simulink model "Proyecto_Final"  (R2017a)
settings: Solver=ode45  StartTime=0.0  StopTime=inf  FixedStep=0.002  RelTol=1e-4
values from neighbouring files (symbols this model uses):
  b_h = b_eq_h * r_h ^ 2 / R_d ^ 2    (= 28800)    [automatas_matlab.m]
  b_t = b_eq_t * r_t ^ 2 / R_w_t ^ 2    (= 27000)    [automatas_matlab.m]
  b_w_h = 30000    [automatas_matlab.m]
  ba_h = M_h * n_h * w_pos_h    (= 172800)    [automatas_matlab.m]
  ba_t = M_t * n_t * w_pos_t    (= 135000)    [automatas_matlab.m]
  bottom_limit_0 = -22    [automatas_matlab.m]
  bottom_limit_1 = -20    [automatas_matlab.m]
  container_vector = [2, 6, 4, 1, 5, 8, 1, 3, 7, 1, 5, 6]    [automatas_matlab.m]    (also in plot_crane.m = [8, 12, 12, 4, 5, 8, 1, 3]; test_traj.m = [8, 5, 9, 4, 5, 8, 4, 6]; test_trajectories.m = [8, 12, 12, 4, 5, 8, 1, 3, 7, 1, 5, 6])
  g = 9.80665    [automatas_matlab.m]
  h_contenedor = 2.79    [automatas_matlab.m]
  K_w_h = 1800000    [automatas_matlab.m]
  Ksa_h = M_h * n_h * w_pos_h^2    (= 207298.578199)    [automatas_matlab.m]
  Ksa_t = M_t * n_t * w_pos_t^2    (= 123542.570499)    [automatas_matlab.m]
  Ksia_h = M_h * w_pos_h ^ 3    (= 82894.8698367)    [automatas_matlab.m]
  Ksia_t = M_t * w_pos_t ^ 3    (= 45223.0125199)    [automatas_matlab.m]
  lambda = 0.91    [automatas_matlab.m]
  left_limit_0 = -32    [automatas_matlab.m]
  left_limit_1 = -30    [automatas_matlab.m]
  M_h = (J_d + J_m_h * r_h ^ 2)/ R_d ^ 2    (= 48014.2222222)    [automatas_matlab.m]
  m_l = 65000    [automatas_matlab.m]
  m_l_min = 15000    [automatas_matlab.m]
  M_t = m_c + (J_w_t + J_m_t * r_t ^ 2)/ R_w_t ^ 2    (= 59008)    [automatas_matlab.m]
  R_d = 0.75    [automatas_matlab.m]
  r_h = 30    [automatas_matlab.m]
  r_t = 15    [automatas_matlab.m]
  R_w_t = 0.5    [automatas_matlab.m]
  right_limit_0 = 52    [automatas_matlab.m]
  right_limit_1 = 50    [automatas_matlab.m]
  top_limit_0 = 42    [automatas_matlab.m]
  top_limit_1 = 40    [automatas_matlab.m]
  v_max_h_load = 1.5    [automatas_matlab.m]
  v_max_h_unload = 3    [automatas_matlab.m]
  v_max_t = 4    [automatas_matlab.m]
  x_t0 = 0    [automatas_matlab.m]
  y_t0 = 45    [automatas_matlab.m]    (also in crane.m; plot_crane.m; plot_crane_test.m)
  yl0 = h_contenedor + 5    (= 7.79)    [automatas_matlab.m]
undefined symbols (not defined in the file or in its folder): DiscIntNeverNeededParam
libraries: simulink x8, vrlib x1, sldrtlib x1
(part 1 of 2)
settings Model: SimulationMode=accelerator  Creator=elust  LastModifiedBy=laure
settings OptimizationCC: UseDivisionForNetSlopeComputation=on  UseFloatMulNetSlope=on  DefaultUnderspecifiedDataType=single  StateBitsets=on  DataBitsets=on  EfficientMapNaN2IntZero=off
settings HardwareCC: TargetBitPerPointer=64  TargetBitPerSizeT=64  TargetBitPerPtrDiffT=64  TargetLongLongMode=on  TargetIntDivRoundTo=Zero  TargetEndianess=LittleEndian  TargetWordSize=64  TargetHWDeviceType=MATLAB Host  ProdEqTarget=off
settings CodeAppCC: MaxIdLength=128
settings GRTTargetCC: TargetLangStandard=C89/C90 (ANSI)  CombineOutputUpdateFcns=off  GRTInterface=on

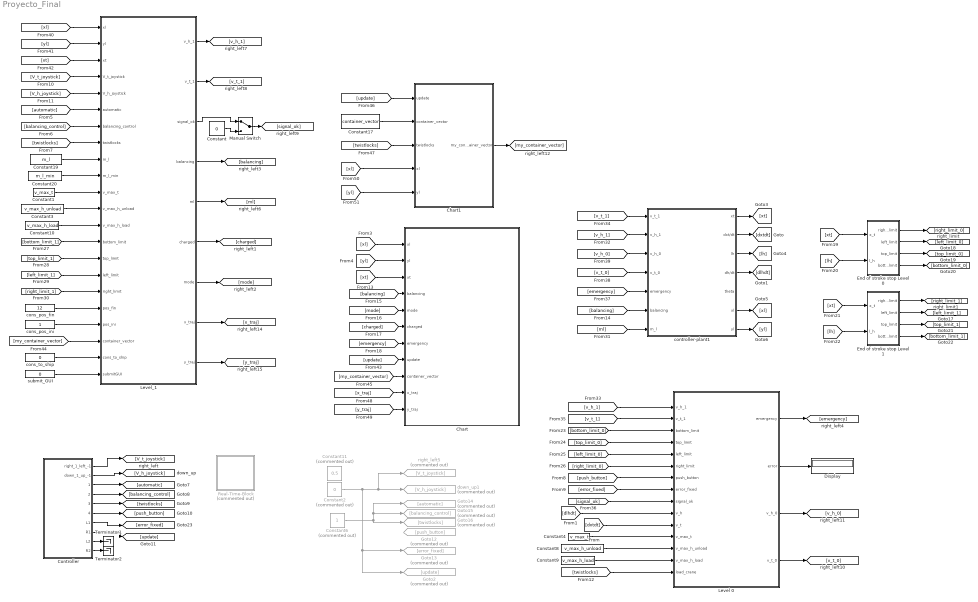
== system Proyecto_Final ==
  Chart : Stateflow chart  TreatAsAtomicUnit=on
  Chart1 : Stateflow chart  TreatAsAtomicUnit=on
  Constant : Constant  Value=0
  Constant1 : Constant  Value=v_max_t
  Constant10 : Constant  Value=v_max_h_load
  Constant11 : Constant  Commented=on  Value=0.5
  Constant17 : Constant  Value=container_vector
  Constant19 : Constant  Value=m_l
  Constant2 : Constant  Commented=on  Value=0
  Constant20 : Constant  Value=m_l_min
  Constant3 : Constant  Value=v_max_h_unload
  Constant4 : Constant  Value=v_max_t
  Constant6 : Constant  Commented=on
  Constant8 : Constant  Value=v_max_h_unload
  Constant9 : Constant  Value=v_max_h_load
  Controller : Subsystem
  Display : Display
  End of stroke stop Level 0 : Subsystem
  End of stroke stop Level 1 : Subsystem
  Goto12 : Goto  Commented=on  GotoTag=push_button
  Goto13 : Goto  Commented=on  GotoTag=error_fixed
  Goto14 : Goto  Commented=on  GotoTag=automatic
  Goto15 : Goto  Commented=on  GotoTag=balancing_control
  Goto16 : Goto  Commented=on  GotoTag=twistlocks
  Goto2 : Goto  Commented=on  GotoTag=update
  Level 0 : Stateflow chart  TreatAsAtomicUnit=on
  "Level_1 " : Stateflow chart  TreatAsAtomicUnit=on
  Manual Switch : ManualSwitch
  Real-Time-Block : Subsystem  Commented=on
  Terminator1 : Terminator
  Terminator2 : Terminator
  cons_pos_fin : Constant  Value=12
  cons_pos_ini : Constant
  cons_to_ship : Constant  Value=0
  controller-plant1 : Subsystem
  down_up1 : Goto  Commented=on  GotoTag=V_h_joystick
  right_left5 : Goto  Commented=on  GotoTag=V_t_joystick
  submit_GUI : Constant  Value=0
  wires:
  Level 0/2(error) -> Display/1
  [push_button] -> Level 0/7(push_button)
  [error_fixed] -> Level 0/8(error_fixed)
  Constant4/1 -> Level 0/12(v_max_t)
  Constant8/1 -> Level 0/13(v_max_h_unload)
  Constant9/1 -> Level 0/14(v_max_h_load)
  [twistlocks] -> Level 0/15(load_crane)
  controller-plant1/2(dxt/dt) -> [dxtdt]
  [dxtdt] -> Level 0/11(v_t)
  [dlhdt] -> Level 0/10(v_h)
  controller-plant1/4(dh/dt) -> [dlhdt]
  controller-plant1/1("xt ") -> [xt]
  controller-plant1/3(lh) -> [lh]
  controller-plant1/6(xl) -> [xl]
  controller-plant1/7(yl) -> [yl]
  Level 0/4(v_t_0) -> [v_t_0]
  Constant/1 -> Manual Switch/2
  "Level_1 "/3(signal_ok) -> Manual Switch/1
  Level 0/1(emergency) -> [emergency]
  Level 0/3(v_h_0) -> [v_h_0]
  Constant19/1 -> "Level_1 "/9(m_l)
  Constant20/1 -> "Level_1 "/10(m_l_min)
  Controller/3(1) -> [automatic]
  Controller/4(2) -> [balancing_control]
  Controller/5(3) -> [twistlocks]
  Controller/6(4) -> [push_button]
  [automatic] -> "Level_1 "/6(automatic)
  [balancing_control] -> "Level_1 "/7(balancing_control)
  [twistlocks] -> "Level_1 "/8(twistlocks)
  Controller/8(R1) -> [update]
  Controller/1(right_1_left_-1) -> [V_t_joystick]
  Controller/2(down_1_up_-1) -> [V_h_joystick]
  Controller/7(L1) -> [error_fixed]
  Controller/9(L2) -> Terminator1/1
  Controller/10(R2) -> Terminator2/1
  [V_t_joystick] -> "Level_1 "/4(V_t_joystick)
  [V_h_joystick] -> "Level_1 "/5(V_h_joystick)
  [yl] -> Chart/2(yl)
  [xl] -> Chart/1(xl)
  Constant1/1 -> "Level_1 "/11(v_max_t)
  Constant3/1 -> "Level_1 "/12(v_max_h_unload)
  Constant10/1 -> "Level_1 "/13(v_max_h_load)
  [xt] -> Chart/3(xt)
  "Level_1 "/7(mode) -> [mode]
  "Level_1 "/6(charged) -> [charged]
  "Level_1 "/4(balancing) -> [balancing]
  [balancing] -> controller-plant1/6(balancing)
  [charged] -> Chart/6(charged)
  [mode] -> Chart/5(mode)
  [balancing] -> Chart/4(balancing)
  [emergency] -> Chart/7(emergency)
  [xt] -> End of stroke stop Level 0/1(x_t)
  [lh] -> End of stroke stop Level 0/2(l_h)
  End of stroke stop Level 0/1(right_limit) -> [right_limit_0]
  End of stroke stop Level 0/2(left_limit) -> [left_limit_0]
  End of stroke stop Level 0/3(top_limit) -> [top_limit_0]
  End of stroke stop Level 0/4(bottom_limit) -> [bottom_limit_0]
  [lh] -> End of stroke stop Level 1/2(l_h)
  [xt] -> End of stroke stop Level 1/1(x_t)
  [right_limit_0] -> Level 0/6(right_limit)
  [left_limit_0] -> Level 0/5(left_limit)
  [top_limit_0] -> Level 0/4(top_limit)
  [bottom_limit_0] -> Level 0/3(bottom_limit)
  End of stroke stop Level 1/4(bottom_limit) -> [bottom_limit_1]
  End of stroke stop Level 1/3(top_limit) -> [top_limit_1]
  End of stroke stop Level 1/2(left_limit) -> [left_limit_1]
  End of stroke stop Level 1/1(right_limit) -> [right_limit_1]
  [bottom_limit_1] -> "Level_1 "/14(bottom_limit)
  [top_limit_1] -> "Level_1 "/15(top_limit)
  [left_limit_1] -> "Level_1 "/16(left_limit)
  [right_limit_1] -> "Level_1 "/17(right_limit)
  "Level_1 "/5(ml) -> [ml]
  [ml] -> controller-plant1/7(m_l)
  [v_h_1] -> controller-plant1/2(v_h_1)
  [v_h_1] -> Level 0/1(v_h_1)
  "Level_1 "/1(v_h_1) -> [v_h_1]
  "Level_1 "/2(v_t_1) -> [v_t_1]
  [v_t_1] -> controller-plant1/1(v_t_1)
  [v_t_1] -> Level 0/2(v_t_1)
  Manual Switch/1 -> [signal_ok]
  [signal_ok] -> Level 0/9(signal_ok)
  [emergency] -> controller-plant1/5(emergency)
  [v_t_0] -> controller-plant1/4(v_t_0)
  [v_h_0] -> controller-plant1/3(v_h_0)
  cons_pos_fin/1 -> "Level_1 "/18(pos_fin)
  cons_pos_ini/1 -> "Level_1 "/19(pos_ini)
  [xt] -> "Level_1 "/3(xt)
  [yl] -> "Level_1 "/2(yl)
  [xl] -> "Level_1 "/1(xl)
  [update] -> Chart/8(update)
  Chart1/1(my_container_vector) -> [my_container_vector]
  Constant17/1 -> Chart1/2(container_vector)
  [my_container_vector] -> "Level_1 "/20(container_vector)
  [my_container_vector] -> Chart/9(container_vector)
  [update] -> Chart1/1(update)
  [twistlocks] -> Chart1/3(twistlocks)
  "Level_1 "/9(y_traj) -> [y_traj]
  "Level_1 "/8(x_traj) -> [x_traj]
  [x_traj] -> Chart/10(x_traj)
  [y_traj] -> Chart/11(y_traj)
  [xl] -> Chart1/4(xl)
  cons_to_ship/1 -> "Level_1 "/21(cons_to_ship)
  submit_GUI/1 -> "Level_1 "/22(submitGUI)
  [yl] -> Chart1/5(yl)
  Constant2/1 -> Goto13/1, Goto2/1, right_left5/1, down_up1/1
  Constant6/1 -> Goto15/1, Goto14/1, Goto16/1

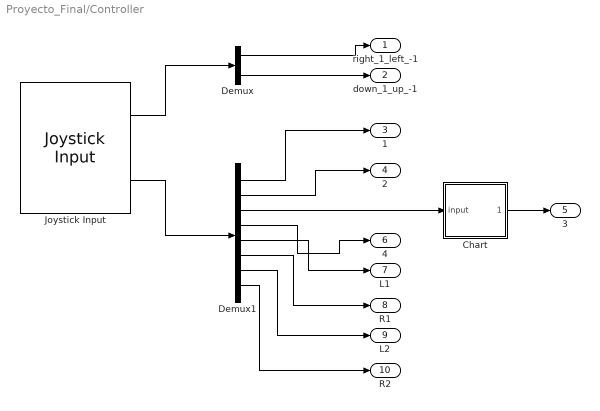
== system Proyecto_Final/Controller ==
  Chart : Stateflow chart  TreatAsAtomicUnit=on
  Demux : Demux  Outputs=2
  Demux1 : Demux  Outputs=8
  Joystick Input : vrlib/Joystick Input  joyid=1  adjustports=on  forcefeed=off
      settings: SourceProductBaseCode=VR
  right_1_left_-1 : Outport
  down_1_up_-1 : Outport  Port=2
  1 : Outport  Port=3
  2 : Outport  Port=4
  3 : Outport  Port=5
  4 : Outport  Port=6
  L1 : Outport  Port=7
  R1 : Outport  Port=8
  L2 : Outport  Port=9
  R2 : Outport  Port=10
  wires:
  Joystick Input/1 -> Demux/1
  Joystick Input/2 -> Demux1/1
  Demux1/1 -> 1/1
  Demux1/2 -> 2/1
  Demux1/8 -> R2/1
  Demux1/5 -> L1/1
  Demux1/4 -> 4/1
  Demux/1 -> right_1_left_-1/1
  Demux1/6 -> R1/1
  Demux1/7 -> L2/1
  Demux/2 -> down_1_up_-1/1
  Demux1/3 -> Chart/1(input)
  Chart/1(output) -> 3/1

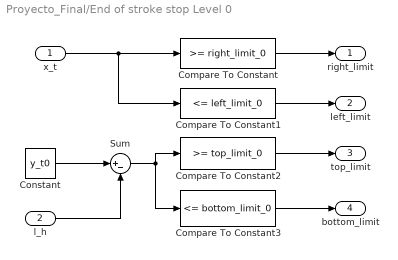
== system Proyecto_Final/End of stroke stop Level 0 ==
  x_t : Inport
  l_h : Inport  Port=2
  Compare To Constant : simulink/Logic and Bit Operations/Compare To Constant  relop=>=  const=right_limit_0  OutDataTypeStr=boolean
  Compare To Constant1 : simulink/Logic and Bit Operations/Compare To Constant  relop=<=  const=left_limit_0  OutDataTypeStr=boolean
  Compare To Constant2 : simulink/Logic and Bit Operations/Compare To Constant  relop=>=  const=top_limit_0  OutDataTypeStr=boolean
  Compare To Constant3 : simulink/Logic and Bit Operations/Compare To Constant  relop=<=  const=bottom_limit_0  OutDataTypeStr=boolean
  Constant : Constant  Value=y_t0
  Sum : Sum  Inputs=|+-
  right_limit : Outport
  left_limit : Outport  Port=2
  top_limit : Outport  Port=3
  bottom_limit : Outport  Port=4
  wires:
  Compare To Constant3/1 -> bottom_limit/1
  Compare To Constant1/1 -> left_limit/1
  Compare To Constant/1 -> right_limit/1
  Compare To Constant2/1 -> top_limit/1
  x_t/1 -> Compare To Constant1/1, Compare To Constant/1
  Constant/1 -> Sum/1
  l_h/1 -> Sum/2
  Sum/1 -> Compare To Constant2/1, Compare To Constant3/1

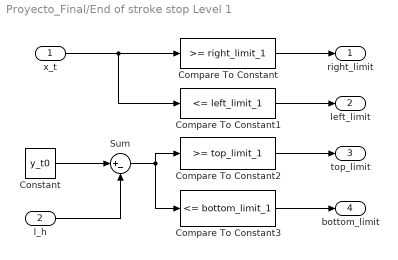
== system Proyecto_Final/End of stroke stop Level 1 ==
  x_t : Inport
  l_h : Inport  Port=2
  Compare To Constant : simulink/Logic and Bit Operations/Compare To Constant  relop=>=  const=right_limit_1  OutDataTypeStr=boolean
  Compare To Constant1 : simulink/Logic and Bit Operations/Compare To Constant  relop=<=  const=left_limit_1  OutDataTypeStr=boolean
  Compare To Constant2 : simulink/Logic and Bit Operations/Compare To Constant  relop=>=  const=top_limit_1  OutDataTypeStr=boolean
  Compare To Constant3 : simulink/Logic and Bit Operations/Compare To Constant  relop=<=  const=bottom_limit_1  OutDataTypeStr=boolean
  Constant : Constant  Value=y_t0
  Sum : Sum  Inputs=|+-
  right_limit : Outport
  left_limit : Outport  Port=2
  top_limit : Outport  Port=3
  bottom_limit : Outport  Port=4
  wires:
  Compare To Constant3/1 -> bottom_limit/1
  Compare To Constant1/1 -> left_limit/1
  Compare To Constant/1 -> right_limit/1
  Compare To Constant2/1 -> top_limit/1
  x_t/1 -> Compare To Constant1/1, Compare To Constant/1
  Constant/1 -> Sum/1
  l_h/1 -> Sum/2
  Sum/1 -> Compare To Constant2/1, Compare To Constant3/1

== system Proyecto_Final/Real-Time-Block ==
  Missed Ticks : Scope
  Real-Time Synchronization : sldrtlib/Real-Time Synchronization  SampleTime=0.1  MaxMissedTicks=10000  ShowMissedTicks=on  YieldWhenWaiting=off
  wires:
  Real-Time Synchronization/1 -> Missed Ticks/1

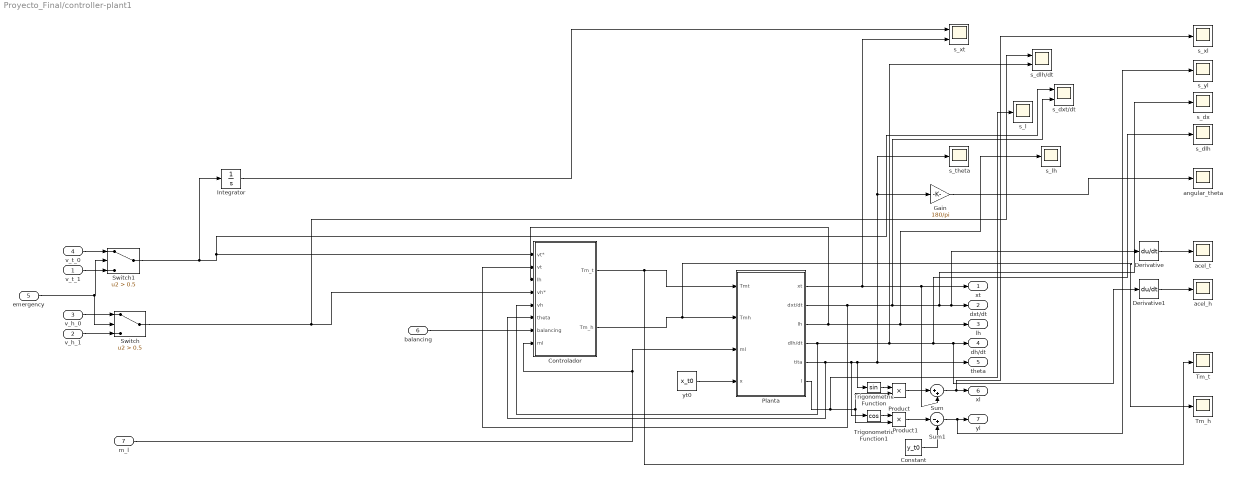
== system Proyecto_Final/controller-plant1 ==
  v_t_1 : Inport
  v_h_1 : Inport  Port=2
  v_h_0 : Inport  Port=3
  v_t_0 : Inport  Port=4
  emergency : Inport  Port=5
  balancing : Inport  Port=6
  m_l : Inport  Port=7
  Constant : Constant  Value=y_t0
  Controlador : Subsystem
  Derivative : Derivative
  Derivative1 : Derivative
  Gain : Gain  Gain=180/pi
  Integrator : Integrator
  Planta : Subsystem
  Product : Product
  Product1 : Product
  Sum : Sum  Inputs=|++
  Sum1 : Sum  Inputs=|-+
  Switch : Switch  Criteria=u2 > Threshold  Threshold=0.5
  Switch1 : Switch  Criteria=u2 > Threshold  Threshold=0.5
  Tm_h : Scope
  "Tm_t " : Scope
  Trigonometric Function : Trigonometry
  Trigonometric Function1 : Trigonometry  Operator=cos
  acel_h : Scope
  acel_t : Scope
  angular_theta : Scope
  s_dlh : Scope
  s_dlh/dt : Scope  NumInputPorts=2
  s_dx : Scope
  s_dxt/dt : Scope  NumInputPorts=2
  s_l : Scope
  s_lh : Scope
  "s_theta " : Scope
  "s_xl " : Scope
  s_xt : Scope  NumInputPorts=2
  "s_yl " : Scope
  yt0 : Constant  Value=x_t0
  "xt " : Outport
  dxt/dt : Outport  Port=2
  lh : Outport  Port=3
  dh/dt : Outport  Port=4
  theta : Outport  Port=5
  xl : Outport  Port=6
  yl : Outport  Port=7
  wires:
  Switch1/1 -> Integrator/1, Controlador/1(vt*), s_dxt/dt/1
  yt0/1 -> Planta/4(x)
  Controlador/1(Tm_t) -> "Tm_t "/1, Planta/1(Tmt)
  Planta/5(tita) -> Controlador/6(theta), Trigonometric Function/1, theta/1, Gain/1, "s_theta "/1, Trigonometric Function1/1
  m_l/1 -> Planta/3(ml), Controlador/8(ml)
  Planta/3(lh) -> Controlador/3(lh), s_lh/1, lh/1
  Switch/1 -> s_dlh/dt/1, Controlador/4(vh*)
  Planta/1(xt) -> s_xt/2, Sum/2, "xt "/1
  Planta/6(l) -> s_l/1, Product/2, Product1/2
  Trigonometric Function1/1 -> Product1/1
  Trigonometric Function/1 -> Product/1
  Sum/1 -> "s_xl "/1, xl/1
  Product/1 -> Sum/1
  Product1/1 -> Sum1/1
  Constant/1 -> Sum1/2
  Integrator/1 -> s_xt/1
  Sum1/1 -> "s_yl "/1, yl/1
  emergency/1 -> Switch/2, Switch1/2
  v_t_1/1 -> Switch1/3
  v_t_0/1 -> Switch1/1
  v_h_0/1 -> Switch/1
  v_h_1/1 -> Switch/3
  balancing/1 -> Controlador/7(balancing)
  Gain/1 -> angular_theta/1
  Planta/4(dlh/dt) -> Controlador/5(vh), s_dlh/1, Derivative1/1, dh/dt/1, s_dlh/dt/2
  Planta/2(dxt/dt) -> Controlador/2(vt), s_dxt/dt/2, s_dx/1, Derivative/1, dxt/dt/1
  Derivative/1 -> acel_t/1
  Derivative1/1 -> acel_h/1
  Controlador/2(Tm_h) -> Tm_h/1, Planta/2(Tmh)

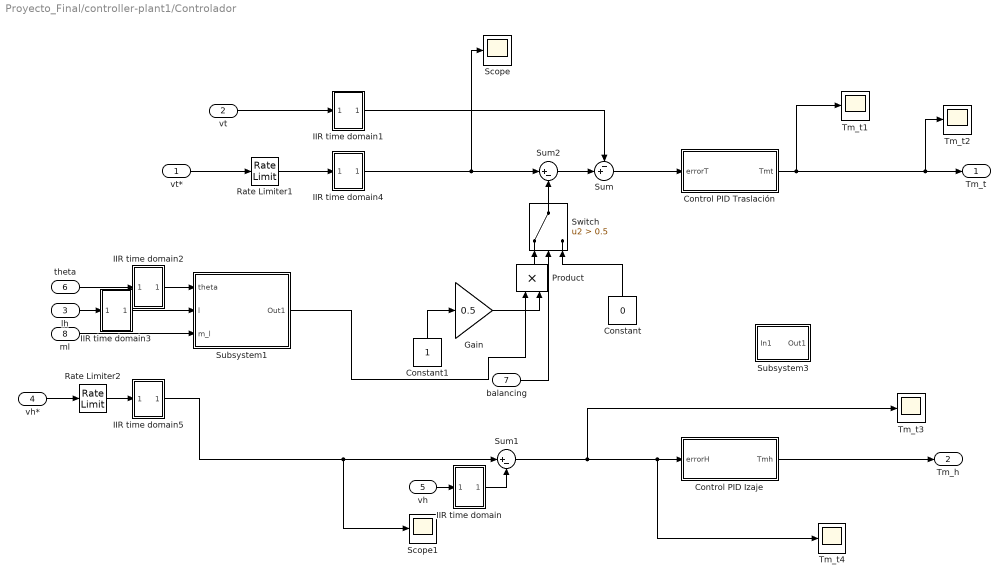
== system Proyecto_Final/controller-plant1/Controlador ==
  vt* : Inport
  vt : Inport  Port=2
  lh : Inport  Port=3
  vh* : Inport  Port=4
  vh : Inport  Port=5
  theta : Inport  Port=6
  balancing : Inport  Port=7
  ml : Inport  Port=8
  Constant : Constant  Value=0
  Constant1 : Constant
  Control PID Izaje : Subsystem
  "Control PID Traslación " : Subsystem
  Gain : Gain  Gain=0.5
  IIR time domain : Subsystem
  IIR time domain1 : Subsystem
  IIR time domain2 : Subsystem
  IIR time domain3 : Subsystem
  IIR time domain4 : Subsystem
  IIR time domain5 : Subsystem
  Product : Product
  Rate Limiter1 : RateLimiter  RisingSlewLimit=0.5  FallingSlewLimit=-0.5  SampleTimeMode=inherited
  Rate Limiter2 : RateLimiter  RisingSlewLimit=0.5  FallingSlewLimit=-0.5  SampleTimeMode=inherited
  Scope : Scope
  Scope1 : Scope
  Subsystem1 : Subsystem
  Subsystem3 : Subsystem
  Sum : Sum  Inputs=-+|
  Sum1 : Sum  Inputs=|+-
  Sum2 : Sum  Inputs=|+-
  Switch : Switch  Criteria=u2 > Threshold  Threshold=0.5
  Tm_t{1..4} (4 alike) : Scope
  Tm_t : Outport
  Tm_h : Outport  Port=2
  wires:
  lh/1 -> IIR time domain3/1(In1)
  vh/1 -> IIR time domain/1(In1)
  Subsystem1/1(Out1) -> Product/1
  theta/1 -> IIR time domain2/1(In1)
  Gain/1 -> Product/2
  vt/1 -> IIR time domain1/1(In1)
  ml/1 -> Subsystem1/3(m_l)
  vh*/1 -> Rate Limiter2/1
  Sum2/1 -> Sum/2
  Switch/1 -> Sum2/2
  Product/1 -> Switch/1
  balancing/1 -> Switch/2
  Constant/1 -> Switch/3
  Constant1/1 -> Gain/1
  vt*/1 -> Rate Limiter1/1
  Sum1/1 -> Tm_t4/1, Control PID Izaje/1(errorH), Tm_t3/1
  Sum/1 -> "Control PID Traslación "/1(errorT)
  "Control PID Traslación "/1(Tmt) -> Tm_t2/1, Tm_t/1, Tm_t1/1
  Control PID Izaje/1(Tmh) -> Tm_h/1
  IIR time domain1/1(Out1) -> Sum/1
  IIR time domain/1(Out1) -> Sum1/2
  IIR time domain2/1(Out1) -> Subsystem1/1(theta)
  IIR time domain3/1(Out1) -> Subsystem1/2(l)
  IIR time domain5/1(Out1) -> Scope1/1, Sum1/1
  IIR time domain4/1(Out1) -> Scope/1, Sum2/1
  Rate Limiter1/1 -> IIR time domain4/1(In1)
  Rate Limiter2/1 -> IIR time domain5/1(In1)

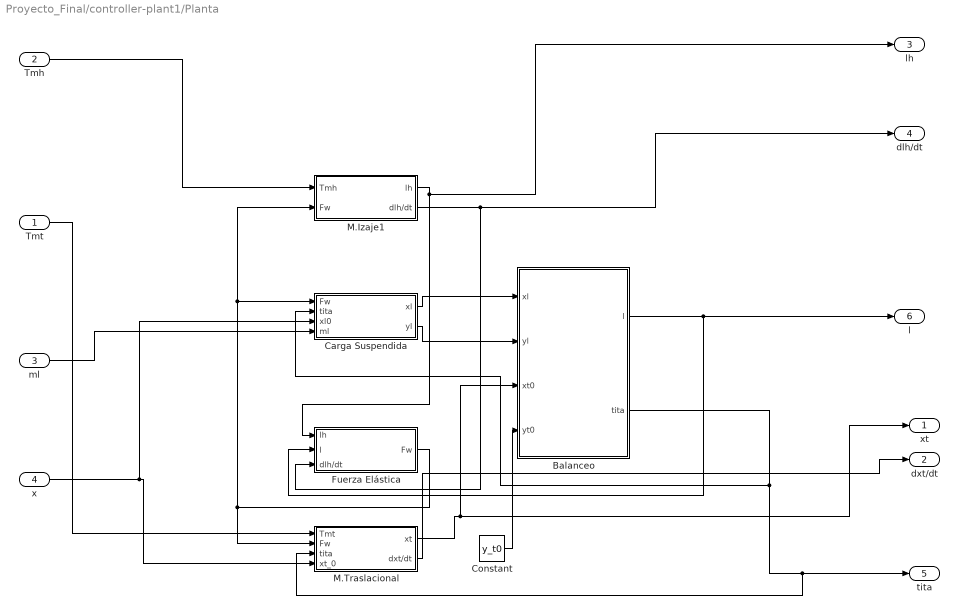
== system Proyecto_Final/controller-plant1/Planta ==
  Tmt : Inport
  Tmh : Inport  Port=2
  ml : Inport  Port=3
  x : Inport  Port=4
  Balanceo : MATLAB Function  TreatAsAtomicUnit=on
  Carga Suspendida : Subsystem
  Constant : Constant  Value=y_t0
  Fuerza Elástica : Subsystem
  M.Izaje1 : Subsystem
  M.Traslacional : Subsystem
  xt : Outport
  dxt/dt : Outport  Port=2
  lh : Outport  Port=3
  dlh/dt : Outport  Port=4
  tita : Outport  Port=5
  l : Outport  Port=6
  wires:
  Balanceo/2(tita) -> Carga Suspendida/2(tita), M.Traslacional/3(tita), tita/1
  Balanceo/1(l) -> Fuerza Elástica/2(l), l/1
  M.Izaje1/2(dlh/dt) -> Fuerza Elástica/3(dlh/dt), dlh/dt/1
  Fuerza Elástica/1(Fw) -> M.Traslacional/2(Fw), Carga Suspendida/1(Fw), M.Izaje1/2(Fw)
  x/1 -> Carga Suspendida/3(xl0), M.Traslacional/4(xt_0)
  ml/1 -> Carga Suspendida/4(ml)
  M.Izaje1/1(lh) -> lh/1, Fuerza Elástica/1(lh)
  Tmh/1 -> M.Izaje1/1(Tmh)
  Tmt/1 -> M.Traslacional/1("Tmt ")
  Carga Suspendida/1(xl) -> Balanceo/1(xl)
  Carga Suspendida/2(yl) -> Balanceo/2(yl)
  M.Traslacional/1(xt) -> Balanceo/3(xt0), xt/1
  M.Traslacional/2(dxt/dt) -> dxt/dt/1
  Constant/1 -> Balanceo/4(yt0)

== system Proyecto_Final/controller-plant1/Controlador/Control PID Izaje ==
  errorH : Inport
  Discrete-Time Integrator1 : DiscreteIntegrator  InitialConditionSetting=State (most efficient)  SampleTime=0.02  ICPrevOutput=DiscIntNeverNeededParam  ICPrevScaledInput=DiscIntNeverNeededParam
  Discrete-Time Integrator2 : DiscreteIntegrator  InitialConditionSetting=State (most efficient)  SampleTime=0.02  ICPrevOutput=DiscIntNeverNeededParam  ICPrevScaledInput=DiscIntNeverNeededParam
  Gain : Gain  Gain=ba_h
  Gain1 : Gain  Gain=Ksia_h
  Gain2 : Gain  Gain=Ksa_h
  Sum : Sum  Inputs=+++
  Tmh : Outport
  wires:
  errorH/1 -> Discrete-Time Integrator1/1, Gain/1
  Gain2/1 -> Sum/2
  Gain1/1 -> Sum/1
  Gain/1 -> Sum/3
  Sum/1 -> Tmh/1
  Discrete-Time Integrator2/1 -> Gain1/1
  Discrete-Time Integrator1/1 -> Discrete-Time Integrator2/1, Gain2/1

== system Proyecto_Final/controller-plant1/Controlador/Control PID Traslación  ==
  errorT : Inport
  Discrete-Time Integrator1 : DiscreteIntegrator  InitialConditionSetting=State (most efficient)  SampleTime=0.02  ICPrevOutput=DiscIntNeverNeededParam  ICPrevScaledInput=DiscIntNeverNeededParam
  Discrete-Time Integrator2 : DiscreteIntegrator  InitialConditionSetting=State (most efficient)  SampleTime=0.02  ICPrevOutput=DiscIntNeverNeededParam  ICPrevScaledInput=DiscIntNeverNeededParam
  Gain : Gain  Gain=ba_t
  Gain1 : Gain  Gain=Ksia_t
  Gain2 : Gain  Gain=Ksa_t
  Sum : Sum  Inputs=+++
  Tmt : Outport
  wires:
  Discrete-Time Integrator2/1 -> Gain1/1
  errorT/1 -> Discrete-Time Integrator1/1, Gain/1
  Gain2/1 -> Sum/2
  Gain1/1 -> Sum/1
  Gain/1 -> Sum/3
  Sum/1 -> Tmt/1
  Discrete-Time Integrator1/1 -> Discrete-Time Integrator2/1, Gain2/1

== system Proyecto_Final/controller-plant1/Controlador/IIR time domain ==
  In1 : Inport
  1-lambda : Constant  Value=1-lambda
  Delay : Delay  DelayLength=1
  Product : Product
  Product1 : Product
  Sum : Sum  Inputs=|++
  lambda : Constant  Value=lambda
  Out1 : Outport
  wires:
  In1/1 -> Product/1
  1-lambda/1 -> Product/2
  Product/1 -> Sum/1
  lambda/1 -> Product1/2
  Sum/1 -> Out1/1, Delay/1
  Delay/1 -> Product1/1
  Product1/1 -> Sum/2

== system Proyecto_Final/controller-plant1/Controlador/IIR time domain1 ==
  In1 : Inport
  1-lambda : Constant  Value=1-lambda
  Delay : Delay  DelayLength=1
  Product : Product
  Product1 : Product
  Sum : Sum  Inputs=|++
  lambda : Constant  Value=lambda
  Out1 : Outport
  wires:
  In1/1 -> Product/1
  1-lambda/1 -> Product/2
  Product/1 -> Sum/1
  lambda/1 -> Product1/2
  Sum/1 -> Out1/1, Delay/1
  Delay/1 -> Product1/1
  Product1/1 -> Sum/2

== system Proyecto_Final/controller-plant1/Controlador/IIR time domain2 ==
  In1 : Inport
  1-lambda : Constant  Value=1-lambda
  Delay : Delay  DelayLength=1
  Product : Product
  Product1 : Product
  Sum : Sum  Inputs=|++
  lambda : Constant  Value=lambda
  Out1 : Outport
  wires:
  In1/1 -> Product/1
  1-lambda/1 -> Product/2
  Product/1 -> Sum/1
  lambda/1 -> Product1/2
  Sum/1 -> Out1/1, Delay/1
  Delay/1 -> Product1/1
  Product1/1 -> Sum/2

== system Proyecto_Final/controller-plant1/Controlador/IIR time domain3 ==
  In1 : Inport
  1-lambda : Constant  Value=1-lambda
  Delay : Delay  DelayLength=1
  Product : Product
  Product1 : Product
  Sum : Sum  Inputs=|++
  lambda : Constant  Value=lambda
  Out1 : Outport
  wires:
  In1/1 -> Product/1
  1-lambda/1 -> Product/2
  Product/1 -> Sum/1
  lambda/1 -> Product1/2
  Sum/1 -> Out1/1, Delay/1
  Delay/1 -> Product1/1
  Product1/1 -> Sum/2

== system Proyecto_Final/controller-plant1/Controlador/IIR time domain4 ==
  In1 : Inport
  1-lambda : Constant  Value=1-lambda
  Delay : Delay  DelayLength=1
  Product : Product
  Product1 : Product
  Sum : Sum  Inputs=|++
  lambda : Constant  Value=lambda
  Out1 : Outport
  wires:
  In1/1 -> Product/1
  1-lambda/1 -> Product/2
  Product/1 -> Sum/1
  lambda/1 -> Product1/2
  Sum/1 -> Out1/1, Delay/1
  Delay/1 -> Product1/1
  Product1/1 -> Sum/2

== system Proyecto_Final/controller-plant1/Controlador/IIR time domain5 ==
  In1 : Inport
  1-lambda : Constant  Value=1-lambda
  Delay : Delay  DelayLength=1
  Product : Product
  Product1 : Product
  Sum : Sum  Inputs=|++
  lambda : Constant  Value=lambda
  Out1 : Outport
  wires:
  In1/1 -> Product/1
  1-lambda/1 -> Product/2
  Product/1 -> Sum/1
  lambda/1 -> Product1/2
  Sum/1 -> Out1/1, Delay/1
  Delay/1 -> Product1/1
  Product1/1 -> Sum/2

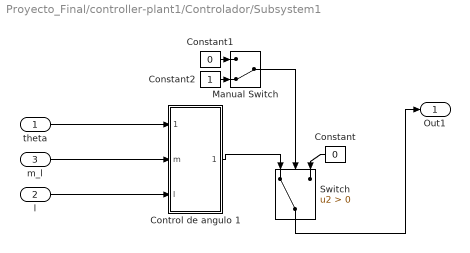
== system Proyecto_Final/controller-plant1/Controlador/Subsystem1 ==
  theta : Inport
  l : Inport  Port=2
  m_l : Inport  Port=3
  Constant : Constant  Value=0
  Constant1 : Constant  Value=0
  Constant2 : Constant
  Control de angulo 1 : Subsystem
  Manual Switch : ManualSwitch  CurrentSetting=0
  Switch : Switch  Criteria=u2 > Threshold
  Out1 : Outport
  wires:
  m_l/1 -> Control de angulo 1/2(m)
  l/1 -> Control de angulo 1/3(l)
  Constant/1 -> Switch/3
  Constant2/1 -> Manual Switch/2
  Control de angulo 1/1(Out1) -> Switch/1
  Manual Switch/1 -> Switch/2
  Constant1/1 -> Manual Switch/1
  theta/1 -> Control de angulo 1/1(theta)
  Switch/1 -> Out1/1

== system Proyecto_Final/controller-plant1/Controlador/Subsystem3 ==
  In1 : Inport
  3 : Gain  Gain=4
  Sum5 : Sum  Inputs=|+-
  dl_h(t)3 : Integrator
  Out1 : Outport
  wires:
  3/1 -> Out1/1, Sum5/2  "VtC_filtrada"
  dl_h(t)3/1 -> 3/1
  Sum5/1 -> dl_h(t)3/1  "FILTROt"
  In1/1 -> Sum5/1

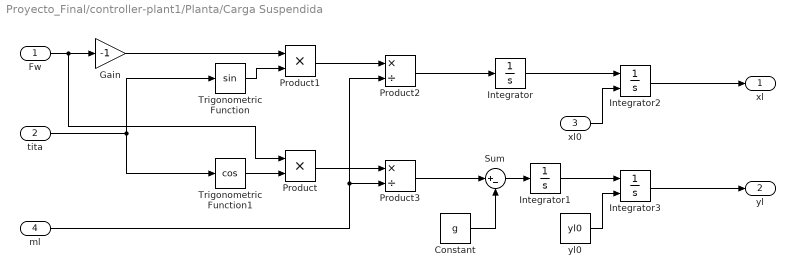
== system Proyecto_Final/controller-plant1/Planta/Carga Suspendida ==
  Fw : Inport
  tita : Inport  Port=2
  xl0 : Inport  Port=3
  ml : Inport  Port=4
  Constant : Constant  Value=g
  Gain : Gain  Gain=-1
  Integrator : Integrator
  Integrator1 : Integrator
  Integrator2 : Integrator  InitialConditionSource=external
  Integrator3 : Integrator  InitialConditionSource=external
  Product : Product
  Product1 : Product
  Product2 : Product  Inputs=*/
  Product3 : Product  Inputs=*/
  Sum : Sum  Inputs=|+-
  Trigonometric Function : Trigonometry
  Trigonometric Function1 : Trigonometry  Operator=cos
  yl0 : Constant  Value=yl0
  xl : Outport
  yl : Outport  Port=2
  wires:
  tita/1 -> Trigonometric Function/1, Trigonometric Function1/1
  Constant/1 -> Sum/2
  Trigonometric Function1/1 -> Product/2
  Fw/1 -> Product/1, Gain/1
  Trigonometric Function/1 -> Product1/2
  Sum/1 -> Integrator1/1
  Integrator/1 -> Integrator2/1
  Integrator1/1 -> Integrator3/1
  yl0/1 -> Integrator3/2
  xl0/1 -> Integrator2/2
  Integrator2/1 -> xl/1
  Integrator3/1 -> yl/1
  Product/1 -> Product3/1
  Product1/1 -> Product2/1
  ml/1 -> Product2/2, Product3/2
  Product2/1 -> Integrator/1
  Product3/1 -> Sum/1
  Gain/1 -> Product1/1

== system Proyecto_Final/controller-plant1/Planta/Fuerza Elástica ==
  lh : Inport
  l : Inport  Port=2
  dlh/dt : Inport  Port=3
  Derivative : Derivative
  Kw : Gain  Gain=K_w_h
  Sum : Sum  Inputs=|-+
  Sum1 : Sum  Inputs=|+-
  Sum2 : Sum
  bw : Gain  Gain=b_w_h
  Fw : Outport
  wires:
  l/1 -> Sum/2, Derivative/1
  lh/1 -> Sum/1
  Sum/1 -> Kw/1
  Derivative/1 -> Sum1/1
  dlh/dt/1 -> Sum1/2
  Sum1/1 -> bw/1
  Sum2/1 -> Fw/1
  Kw/1 -> Sum2/1
  bw/1 -> Sum2/2

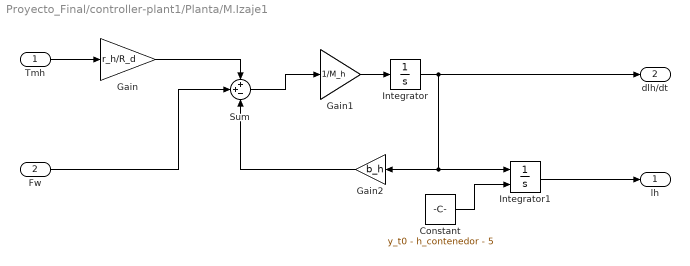
== system Proyecto_Final/controller-plant1/Planta/M.Izaje1 ==
  Tmh : Inport
  Fw : Inport  Port=2
  Constant : Constant  Value=y_t0 - h_contenedor - 5
  Gain : Gain  Gain=r_h/R_d
  Gain1 : Gain  Gain=1/M_h
  Gain2 : Gain  Gain=b_h
  Integrator : Integrator
  Integrator1 : Integrator  InitialConditionSource=external
  Sum : Sum  Inputs=++-
  lh : Outport
  dlh/dt : Outport  Port=2
  wires:
  Tmh/1 -> Gain/1
  Gain/1 -> Sum/1
  Sum/1 -> Gain1/1
  Gain1/1 -> Integrator/1
  Integrator/1 -> dlh/dt/1, Integrator1/1, Gain2/1
  Gain2/1 -> Sum/3
  Fw/1 -> Sum/2
  Constant/1 -> Integrator1/2
  Integrator1/1 -> lh/1

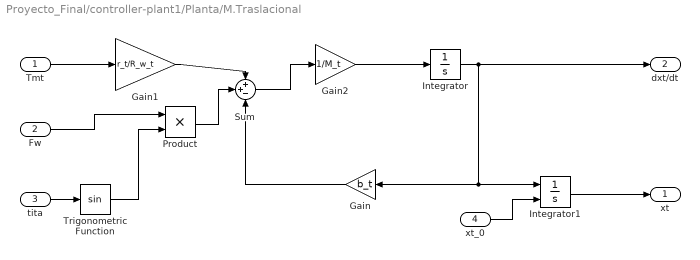
== system Proyecto_Final/controller-plant1/Planta/M.Traslacional ==
  "Tmt " : Inport
  Fw : Inport  Port=2
  tita : Inport  Port=3
  xt_0 : Inport  Port=4
  Gain : Gain  Gain=b_t
  Gain1 : Gain  Gain=r_t/R_w_t
  Gain2 : Gain  Gain=1/M_t
  Integrator : Integrator
  Integrator1 : Integrator  InitialConditionSource=external
  Product : Product
  Sum : Sum  Inputs=++-
  Trigonometric Function : Trigonometry
  xt : Outport
  dxt/dt : Outport  Port=2
  wires:
  Gain2/1 -> Integrator/1
  Trigonometric Function/1 -> Product/2
  tita/1 -> Trigonometric Function/1
  Integrator/1 -> dxt/dt/1, Integrator1/1, Gain/1
  Gain/1 -> Sum/3
  Fw/1 -> Product/1
  Product/1 -> Sum/2
  Sum/1 -> Gain2/1
  Gain1/1 -> Sum/1
  xt_0/1 -> Integrator1/2
  "Tmt "/1 -> Gain1/1
  Integrator1/1 -> xt/1

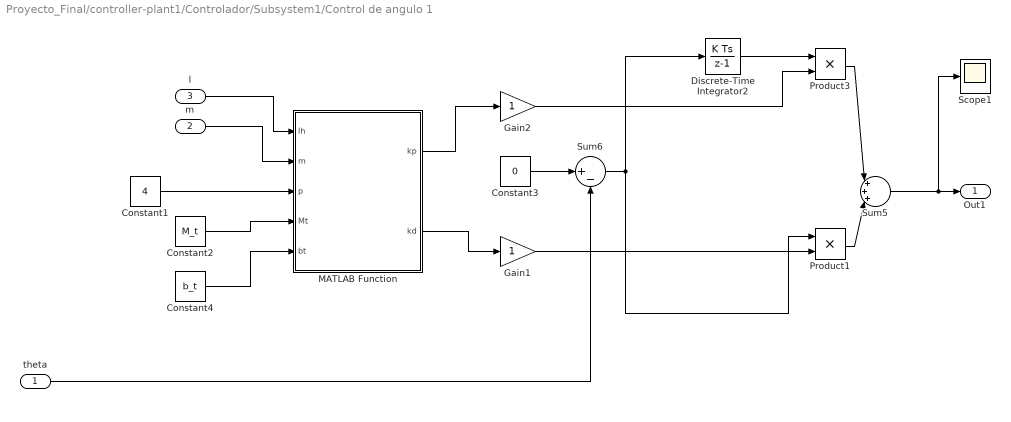
== system Proyecto_Final/controller-plant1/Controlador/Subsystem1/Control de angulo 1 ==
  theta : Inport
  m : Inport  Port=2
  l : Inport  Port=3
  Constant1 : Constant  Value=4
  Constant2 : Constant  Value=M_t
  Constant3 : Constant  Value=0
  Constant4 : Constant  Value=b_t
  Discrete-Time Integrator2 : DiscreteIntegrator  InitialConditionSetting=State (most efficient)  SampleTime=0.02  ICPrevOutput=DiscIntNeverNeededParam  ICPrevScaledInput=DiscIntNeverNeededParam
  Gain1 : Gain
  Gain2 : Gain
  MATLAB Function : MATLAB Function  TreatAsAtomicUnit=on
  Product1 : Product
  Product3 : Product
  Scope1 : Scope
  Sum5 : Sum  Inputs=|+++|
  Sum6 : Sum  Inputs=|+-
  Out1 : Outport
  wires:
  Product1/1 -> Sum5/3
  Sum5/1 -> Scope1/1, Out1/1
  m/1 -> MATLAB Function/2(m)
  l/1 -> MATLAB Function/1(lh)
  Constant2/1 -> MATLAB Function/4(Mt)
  Constant4/1 -> MATLAB Function/5(bt)
  Sum6/1 -> Product1/1, Discrete-Time Integrator2/1
  Product3/1 -> Sum5/1
  theta/1 -> Sum6/2
  Constant3/1 -> Sum6/1
  MATLAB Function/1(kp) -> Gain2/1
  MATLAB Function/2(kd) -> Gain1/1
  Gain1/1 -> Product1/2
  Gain2/1 -> Product3/2
  Discrete-Time Integrator2/1 -> Product3/1
  Constant1/1 -> MATLAB Function/3(p)

== stateflow chart Proyecto_Final/Chart1 ==
  state containers
    entry:
    aux_container_vector = zeros(length(container_vector), 1);
    during:
    state Normal [parallel]
      settings: executionOrder=1
      state Wait
        entry:
        my_container_vector = container_vector + aux_container_vector;
      state update_containers
        entry:
        update_container_vector()
      (default) -> Wait
      Wait -> update_containers : [update == 1  && after(1, sec)]
      update_containers -> Wait : [update == 0 && after(0.1,sec) ]
    state Spreader [parallel]
      settings: executionOrder=2
      state Unchaged
        during:
        charged = 0;
      state Charged
        during:
        charged = 1;
      (default) -> Charged
      Charged -> Unchaged : [twistlocks == 0]
      Unchaged -> Charged : [twistlocks == 1]
  data: update input; container_vector input; aux_container_vector local; component local; my_container_vector output; twistlocks input; charged local; xl input; yl input
  function update_container_vector:
    | function update_container_vector()
    | 
    | 
    | x_edge = 2;
    | y_edge = 2;
    | container_size_x = 2.44;
    | container_size_y = 2.79;
    | y_ini = 4;
    | y_platform = 0;
    | y_ship_botton = -10;
    | 
    | y_safe = 2;
    | 
    | position_vector = zeros(length(my_container_vector));
    | for i = 1:length(my_container_vector)
    |     position_vector(i) = i;
    | end
    | 
    | x_ini = 0;
    | y_fin = 0;
    | x_positions = position_vector * container_size_x - container_size_x / 2 + x_edge;
    | 
    | my_ini = 0;
    | my_fin = 0;
    | if xl > 0
    |     if xl > x_positions(length(x_positions))
    |         my_fin = length(x_positions);
    |     else
    |         for i = 1:length(x_positions)
    |             if xl > x_positions(i) - container_size_x / 2 && xl < x_positions(i) + container_size_x / 2
    |                 my_fin = i;
    |                 break;
    |             end
    |         end
    |     end
    | end
    |         
    | 
    | 
    | 
    | component = my_fin;
    | 
    | 
    | if my_fin ~= 0
    |     if yl < (container_size_y * my_container_vector(i) + y_ship_botton + container_size_y + 1)
    |         if charged == 1
    |            aux_container_vector(component) = aux_container_vector(component)  + 1;
    |         else
    |           if (my_container_vector(component) ~= 0)
    |               aux_container_vector(component) = aux_container_vector(component)  - 1;
    |            end
    |         end
    |     end
    | end

== stateflow chart Proyecto_Final/Level 0 ==
  settings: updateMethod=DISCRETE  sampleTime=0.02
  state Level0
    state Emergency_limit_switch_horizontal
      entry:
      emergency = 1;
      if (right_limit == 1)
      error = 1;
      else
      error = 2;
      end
    state Normal_Operation
      entry:
      ok = 1;
      iterations = 0;
      max_tol = 10;
      counter = 0;
      during:
      state Normal [parallel]
        entry:
        emergency = 0;
        error = 0;
        if (load_crane == 0)
        v_max_h = v_max_h_unload;
        else
        v_max_h = v_max_h_load;
        end
        during:
        v_t_0 = v_t_1;
        v_h_0 = v_h_1;
        settings: executionOrder=1
      state Signals [parallel]
        settings: executionOrder=2
        state wait
          entry: iterations = iterations + 1;
        state verify
          entry:
          if iterations > 100
          counter = 0;
          iterations= 0;
          end
          counter = counter + 2*( signal_ok - 0.5);
          if (abs(counter) > max_tol)
          ok = 0;
          end
        wait -> verify : after(0.1, sec)
        verify -> wait : after(0.1, sec)
      (default) -> wait
    state Emergency_limit_switch_vertical
      entry:
      emergency = 1;
      if (bottom_limit == 1)
      error = 3;
      else
      error = 4;
      end
    state Emergency_overspeed
      entry:
      emergency = 1;
      error = 5;
    state Emergency_button
      entry:
      emergency = 1;
      error = 6;
    state Emergency_level_1
      entry:
      emergency = 1;
      error = 8;
    (default) -> Normal_Operation
    Normal_Operation -> Emergency_limit_switch_horizontal [order 1] : [(right_limit == 1)||(left_limit == 1)]
    Normal_Operation -> Emergency_limit_switch_vertical [order 3] : [(top_limit == 1) || (bottom_limit == 1)]
    Normal_Operation -> Emergency_overspeed [order 4] : [ (v_t > 1.1 * abs(v_max_t)) || (v_h > 1.1 *abs(v_max_h))]
    Normal_Operation -> Emergency_button [order 5] : [push_button == 1]
    Normal_Operation -> Emergency_level_1 [order 2] : [ok == 0]
  state Emergency
    state emergency_handler
      during:
      [v_t_0, v_h_0] = handleError(error);
    state end_emergency
      entry:
      emergency = 0;
      error = 0;
    (default) -> emergency_handler
    emergency_handler -> end_emergency : [error_fixed == 1]
  (default) -> Level0
  Level0 -> Emergency : [emergency == 1]
  Emergency -> Level0 : [emergency == 0]
  data: my_error function_input; v_t_o function_output; v_h_o function_output; v_h_1 input; v_t_1 input; emergency output; bottom_limit input; top_limit input; left_limit input; right_limit input; push_button input; error_fixed input; signal_ok input; error output; v_h input; v_t input; v_max_t input double; v_max_h_unload input; v_max_h_load input; v_max_h local double; load_crane input; v_h_0 output; v_t_0 output; ok local; counter local; iterations local; max_tol local
  function [v_t_o, v_h_o] = handleError(my_error):
    | function [v_t_o, v_h_o] = handleError(my_error)
    | v_t_o = v_t_1;
    | v_h_o = v_h_1;
    | if (my_error == 1) || (my_error == 2) % Right and left
    |     v_t_o = 0;
    | elseif (my_error == 3) || (my_error == 4) % Botton and top
    |     v_h_o = 0;
    | elseif (my_error == 5) % Overspeed
    |     v_t_o = 0;
    |     v_h_o = 0;
    | elseif (my_error == 6) % Emergency button
    |     v_t_o = 0;
    |     v_h_o = 0;
    | elseif (my_error == 7) % Emergency angle
    |     v_h_o = 0;
    |     v_t_o = 0;
    | elseif (my_error == 8) % Emergency level 1
    |     v_h_o = 0;
    |     v_t_o = 0;
    | end
    | end
